simulink model "dynamicPMSM"  (R2023b)
settings: Solver=VariableStepAuto  StartTime=0.0  StopTime=15  RelTol=1e-3
undefined symbols (not defined in the file): B, J, lambda, Ld, Lq, P, R
settings Model: Creator=Akaashdeep B  LastModifiedBy=Akaashdeep B

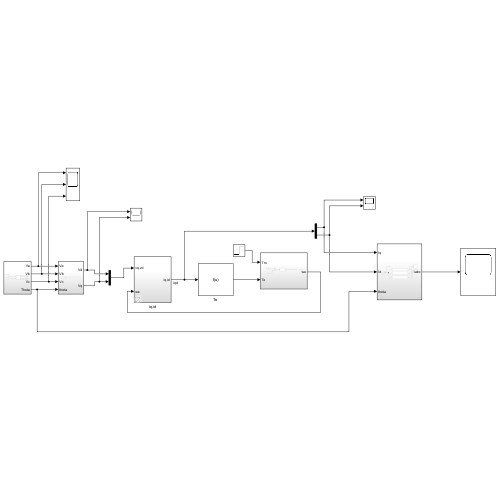
[thumbnail: Simulink's stored preview of the top-level diagram]
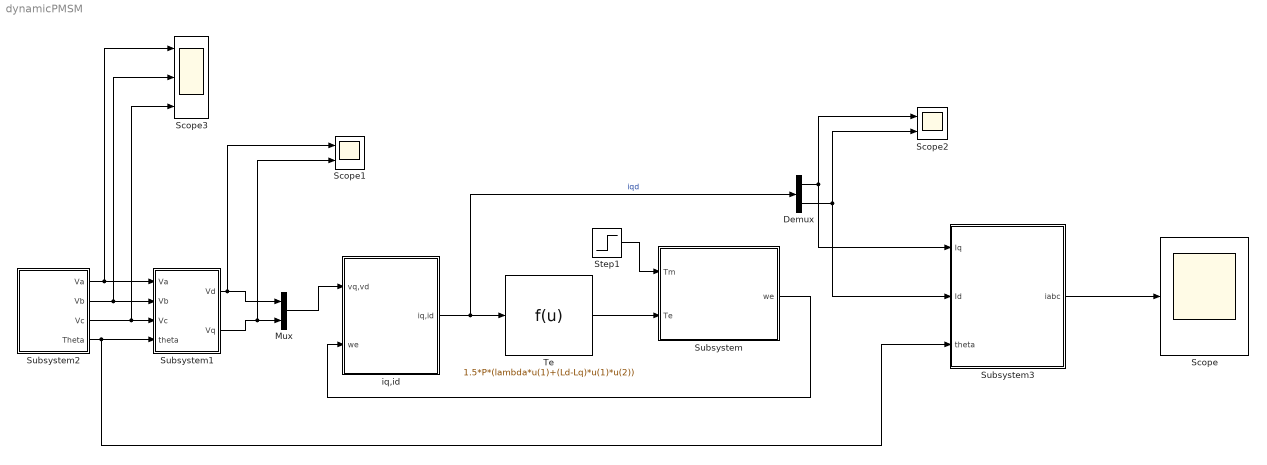
== system dynamicPMSM ==
  Demux : Demux  Outputs=2
  Mux : Mux  Inputs=2
  Scope : Scope
  Scope1 : Scope  NumInputPorts=2
  Scope2 : Scope  NumInputPorts=2
  Scope3 : Scope  NumInputPorts=3
  Step1 : Step  Time=0.1  SampleTime=0
  Subsystem : Subsystem
  Subsystem1 : Subsystem
  Subsystem2 : Subsystem
  Subsystem3 : Subsystem
  "Te " : Fcn  Expr=1.5*P*(lambda*u(1)+(Ld-Lq)*u(1)*u(2))
  iq,id : Subsystem  AncestorBlock=spsPMSynchronousMachineModel/Continuous/iq,id
  wires:
  Subsystem2/4(Theta) -> Subsystem3/3(theta), Subsystem1/4(theta)
  Subsystem2/3(Vc) -> Scope3/3, Subsystem1/3(Vc)
  Subsystem1/2(Vq) -> Scope1/2, Mux/2
  Subsystem2/2(Vb) -> Scope3/2, Subsystem1/2(Vb)
  Subsystem2/1(Va) -> Scope3/1, Subsystem1/1(Va)
  Subsystem1/1(Vd) -> Scope1/1, Mux/1
  Mux/1 -> iq,id/1(vq,vd)
  iq,id/1(iq,id) -> Demux/1, "Te "/1  "iqd"
  Subsystem/1(we) -> iq,id/2(we)
  "Te "/1 -> Subsystem/2(Te)
  Step1/1 -> Subsystem/1(Tm)
  Demux/1 -> Scope2/1, Subsystem3/1(Iq)
  Demux/2 -> Scope2/2, Subsystem3/2(Id)
  Subsystem3/1(iabc) -> Scope/1

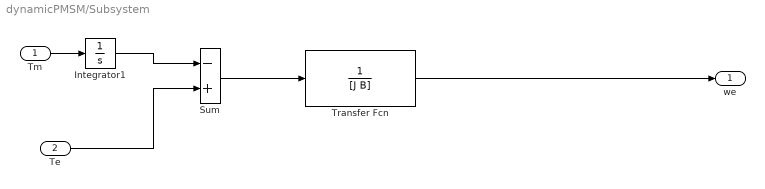
== system dynamicPMSM/Subsystem ==
  Tm : Inport
  Te : Inport  Port=2
  Integrator1 : Integrator
  Sum : Sum  Inputs=-+  InputSameDT=on  SaturateOnIntegerOverflow=on  OutDataTypeStr=Inherit: Same as first input
  Transfer Fcn : TransferFcn  Denominator=[J B]
  we : Outport
  wires:
  Tm/1 -> Integrator1/1
  Sum/1 -> Transfer Fcn/1
  Te/1 -> Sum/2
  Integrator1/1 -> Sum/1
  Transfer Fcn/1 -> we/1

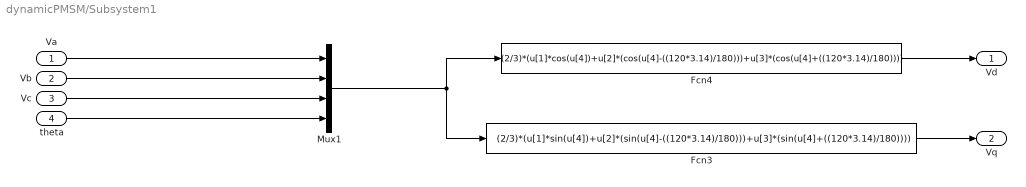
== system dynamicPMSM/Subsystem1 ==
  Va : Inport
  Vb : Inport  Port=2
  Vc : Inport  Port=3
  theta : Inport  Port=4
  Fcn3 : Fcn  Expr=(2/3)*(u[1]*sin(u[4])+u[2]*(sin(u[4]-((120*3.14)/180)))+u[3]*(sin(u[4]+((120*3.14)/180))))
  Fcn4 : Fcn  Expr=(2/3)*(u[1]*cos(u[4])+u[2]*(cos(u[4]-((120*3.14)/180)))+u[3]*(cos(u[4]+((120*3.14)/180))))
  Mux1 : Mux
  Vd : Outport
  Vq : Outport  Port=2
  wires:
  Va/1 -> Mux1/1
  Vb/1 -> Mux1/2
  Mux1/1 -> Fcn3/1, Fcn4/1
  theta/1 -> Mux1/4
  Fcn4/1 -> Vd/1
  Vc/1 -> Mux1/3
  Fcn3/1 -> Vq/1

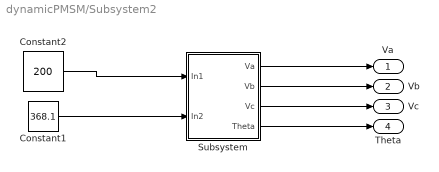
== system dynamicPMSM/Subsystem2 ==
  Constant1 : Constant  Value=368.1
  Constant2 : Constant  Value=200
  Subsystem : Subsystem
  Va : Outport
  Vb : Outport  Port=2
  Vc : Outport  Port=3
  Theta : Outport  Port=4
  wires:
  Constant1/1 -> Subsystem/2(In2)
  Constant2/1 -> Subsystem/1(In1)
  Subsystem/2(Vb) -> Vb/1
  Subsystem/3(Vc) -> Vc/1
  Subsystem/4(Theta) -> Theta/1
  Subsystem/1(Va) -> Va/1

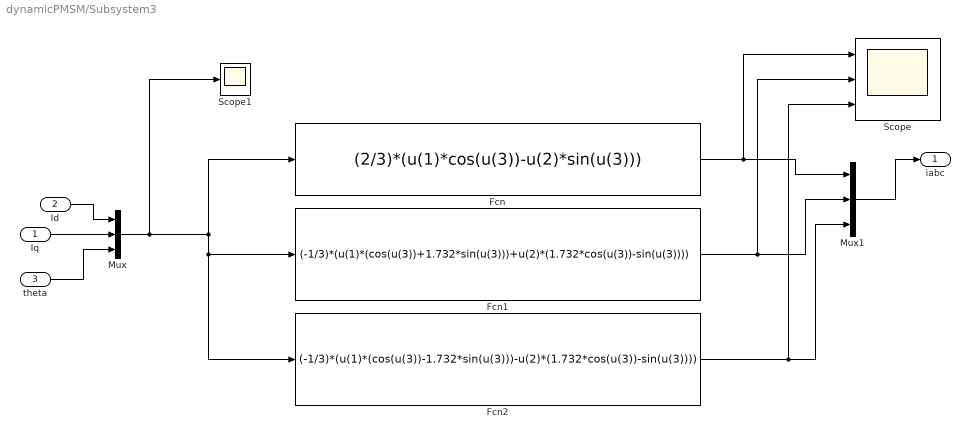
== system dynamicPMSM/Subsystem3 ==
  Iq : Inport
  Id : Inport  Port=2
  theta : Inport  Port=3
  Fcn : Fcn  Expr=(2/3)*(u(1)*cos(u(3))-u(2)*sin(u(3)))
  Fcn1 : Fcn  Expr=(-1/3)*(u(1)*(cos(u(3))+1.732*sin(u(3)))+u(2)*(1.732*cos(u(3))-sin(u(3))))
  Fcn2 : Fcn  Expr=(-1/3)*(u(1)*(cos(u(3))-1.732*sin(u(3)))-u(2)*(1.732*cos(u(3))-sin(u(3))))
  Mux : Mux  Inputs=3
  Mux1 : Mux  Inputs=3
  Scope : Scope  NumInputPorts=3
  Scope1 : Scope
  iabc : Outport
  wires:
  Fcn1/1 -> Scope/2, Mux1/2
  Fcn2/1 -> Scope/3, Mux1/3
  Fcn/1 -> Scope/1, Mux1/1
  Iq/1 -> Mux/2
  Id/1 -> Mux/1
  theta/1 -> Mux/3
  Mux/1 -> Scope1/1, Fcn/1, Fcn2/1, Fcn1/1
  Mux1/1 -> iabc/1

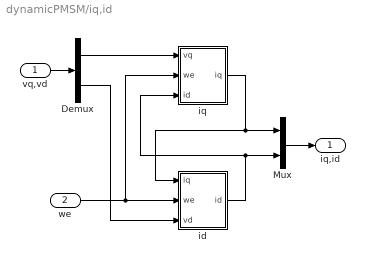
== system dynamicPMSM/iq,id ==
  vq,vd : Inport
  we : Inport  Port=2
  Demux : Demux  Outputs=2
  Mux : Mux  Inputs=2
  id : Subsystem
  iq : Subsystem
  iq,id : Outport  InitialOutput=0  VectorParamsAs1DForOutWhenUnconnected=off
  wires:
  Mux/1 -> iq,id/1
  vq,vd/1 -> Demux/1
  Demux/1 -> iq/1(vq)
  Demux/2 -> id/3(vd)
  iq/1(iq) -> id/1(iq), Mux/1
  we/1 -> id/2(we), iq/2(we)
  id/1(id) -> iq/3(id), Mux/2

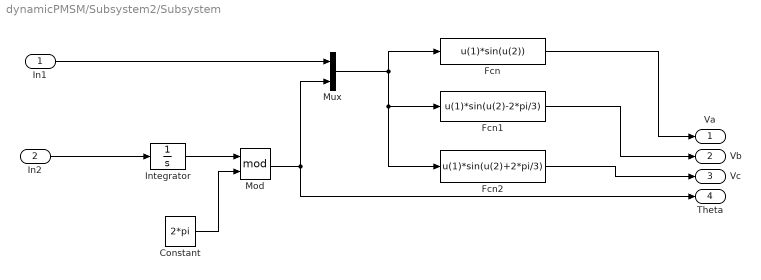
== system dynamicPMSM/Subsystem2/Subsystem ==
  In1 : Inport
  In2 : Inport  Port=2
  Constant : Constant  Value=2*pi
  Fcn : Fcn  Expr=u(1)*sin(u(2))
  Fcn1 : Fcn  Expr=u(1)*sin(u(2)-2*pi/3)
  Fcn2 : Fcn  Expr=u(1)*sin(u(2)+2*pi/3)
  Integrator : Integrator
  Mod : Math  Operator=mod
  Mux : Mux  Inputs=2
  Va : Outport
  Vb : Outport  Port=2
  Vc : Outport  Port=3
  Theta : Outport  Port=4
  wires:
  Mod/1 -> Theta/1, Mux/2
  Constant/1 -> Mod/2
  Mux/1 -> Fcn2/1, Fcn1/1, Fcn/1
  Fcn1/1 -> Vb/1
  Integrator/1 -> Mod/1
  Fcn/1 -> Va/1
  In1/1 -> Mux/1
  Fcn2/1 -> Vc/1
  In2/1 -> Integrator/1

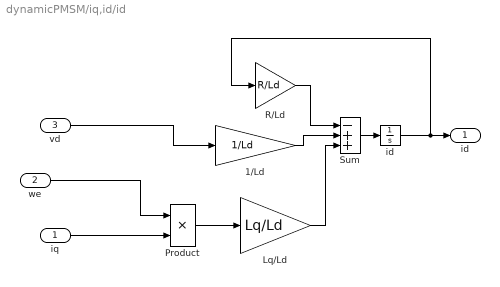
== system dynamicPMSM/iq,id/id ==
  iq : Inport
  we : Inport  Port=2
  vd : Inport  Port=3
  1/Ld : Gain  Gain=1/Ld  SaturateOnIntegerOverflow=on  OutDataTypeStr=Inherit: Same as input  ParamDataTypeStr=Inherit: Same as input
  Lq/Ld : Gain  Gain=Lq/Ld  SaturateOnIntegerOverflow=on  OutDataTypeStr=Inherit: Same as input  ParamDataTypeStr=Inherit: Same as input
  Product : Product  InputSameDT=on  SaturateOnIntegerOverflow=on  OutDataTypeStr=Inherit: Same as first input
  R/Ld : Gain  Gain=R/Ld  SaturateOnIntegerOverflow=on  OutDataTypeStr=Inherit: Same as input  ParamDataTypeStr=Inherit: Same as input
  Sum : Sum  Inputs=-++  InputSameDT=on  SaturateOnIntegerOverflow=on  OutDataTypeStr=Inherit: Same as first input
  "id " : Integrator
  id : Outport  InitialOutput=0  VectorParamsAs1DForOutWhenUnconnected=off
  wires:
  1/Ld/1 -> Sum/2
  R/Ld/1 -> Sum/1
  Lq/Ld/1 -> Sum/3
  Sum/1 -> "id "/1
  Product/1 -> Lq/Ld/1
  "id "/1 -> R/Ld/1, id/1
  vd/1 -> 1/Ld/1
  we/1 -> Product/1
  iq/1 -> Product/2

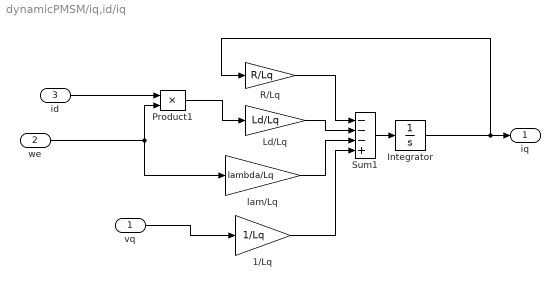
== system dynamicPMSM/iq,id/iq ==
  vq : Inport
  we : Inport  Port=2
  id : Inport  Port=3
  1/Lq : Gain  Gain=1/Lq  SaturateOnIntegerOverflow=on  OutDataTypeStr=Inherit: Same as input  ParamDataTypeStr=Inherit: Same as input
  Integrator : Integrator
  Ld/Lq : Gain  Gain=Ld/Lq  SaturateOnIntegerOverflow=on  OutDataTypeStr=Inherit: Same as input  ParamDataTypeStr=Inherit: Same as input
  Product1 : Product  InputSameDT=on  SaturateOnIntegerOverflow=on  OutDataTypeStr=Inherit: Same as first input
  R/Lq : Gain  Gain=R/Lq  SaturateOnIntegerOverflow=on  OutDataTypeStr=Inherit: Same as input  ParamDataTypeStr=Inherit: Same as input
  Sum1 : Sum  Inputs=---+  InputSameDT=on  SaturateOnIntegerOverflow=on  OutDataTypeStr=Inherit: Same as first input
  lam/Lq : Gain  Gain=lambda/Lq  SaturateOnIntegerOverflow=on  OutDataTypeStr=Inherit: Same as input  ParamDataTypeStr=Inherit: Same as input
  iq : Outport  InitialOutput=0  VectorParamsAs1DForOutWhenUnconnected=off
  wires:
  R/Lq/1 -> Sum1/1
  Ld/Lq/1 -> Sum1/2
  lam/Lq/1 -> Sum1/3
  Sum1/1 -> Integrator/1
  Product1/1 -> Ld/Lq/1
  1/Lq/1 -> Sum1/4
  id/1 -> Product1/1
  vq/1 -> 1/Lq/1
  we/1 -> lam/Lq/1, Product1/2
  Integrator/1 -> R/Lq/1, iq/1
